simulink model "acceleration_generator"  (R2012b)
settings: Solver=ode45  StartTime=0.0  StopTime=10.0  RelTol=1e-3
settings Model: Creator=mchusr  LastModifiedBy=mchusr

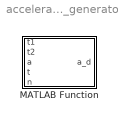
== system acceleration_generator ==
  MATLAB Function : MATLAB Function  TreatAsAtomicUnit=on

== matlab function acceleration_generator/MATLAB Function ==
  data: t1 input; a_d output; t2 input; a input; t input; n input
function a_d = fcn(t1, t2, a, t, n)

T = 4*t1;

for m=1:n
    






end
